simulink model "ProposedProblem2"  (R2013a)
settings: Solver=ode45  StartTime=0.0  StopTime=28800  RelTol=1e-3
undefined symbols (not defined in the file): des, gcbh
settings Model: Creator=gabig  LastModifiedBy=gabig

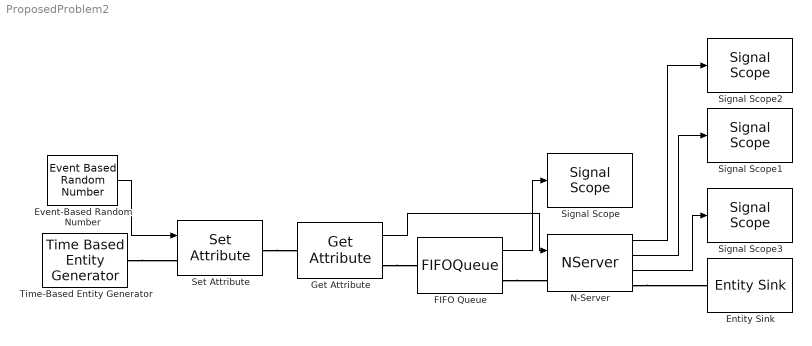
== system ProposedProblem2 ==
  Entity Sink : EntitySink
  Event-Based Random Number : EventBasedRandomNumber  Distribution=Uniform  minUnif=48  maxUnif=72  Seed=12346
  FIFO Queue : FIFOQueue  StatAverageWait=on
      settings: OutputPortMap=o2
  Get Attribute : GetAttribute  AttributeName=Call  EvaluatedDefaultAttributeValue={ []}
      settings: OutputPortMap=o1
  N-Server : NServer  ServiceTimeFrom=Signal port t  StatNumberInBlock=on  StatAverageWait=on  StatUtilization=on
      settings: OutputPortMap=o1,o4,o5
  Set Attribute : SetAttribute  AttributeName=Call  AttributeFrom=Signal port  EvaluatedAttributeValue={ []}
  Signal Scope{,1..3} (4 alike) : SignalScope  LoadFcn=des.scope.CallbackSupport('seLoadFcn',gcbh)  StartFcn=des.scope.CallbackSupport('seStartFcn',gcbh)  StopFcn=des.scope.CallbackSupport('seStopFcn',gcbh)
      settings: CopyFcn=des.scope.CallbackSupport('seCopyFcn',gcbh)  DeleteFcn=des.scope.CallbackSupport('seDeleteFcn',gcbh)  PreSaveFcn=des.scope.CallbackSupport('sePreSaveFcn',gcbh)  NameChangeFcn=des.scope.CallbackSupport('seNameChangeFcn',gcbh)  OpenFcn=des.scope.CallbackSupport('seOpenFcn',gcbh)
  Time-Based Entity Generator : TimeBasedEntityGenerator  Distribution=Exponential  Mean=12
  wires:
  FIFO Queue/1 -> Signal Scope/1
  N-Server/2 -> Signal Scope1/1
  Get Attribute/1 -> N-Server/1
  Event-Based Random Number/1 -> Set Attribute/1
  N-Server/3 -> Signal Scope3/1
  N-Server/1 -> Signal Scope2/1
  connections:
  Get Attribute/RConn1 -- FIFO Queue/LConn1
  Set Attribute/RConn1 -- Get Attribute/LConn1
  Time-Based Entity Generator/RConn1 -- Set Attribute/LConn1
  FIFO Queue/RConn1 -- N-Server/LConn1
  N-Server/RConn1 -- Entity Sink/LConn1
